simulink model "oving2"  (R2024b)
settings: Solver=ode2  StartTime=0.0  StopTime=100  FixedStep=0.01  RelTol=1e-9  AbsTol=1e-9
values from neighbouring files (symbols this model uses):
  U = 0.5    [oving2_data.m]
  w = 0.3    [oving2_data.m]
  w1 = 0.3    [oving2_data.m]
  w2 = 0.55    [oving2_data.m]
  w3 = 0.8    [oving2_data.m]
undefined symbols (not defined in the file or in its folder): a, b, c, d, f, g, h, i, j, k, l, m, n, o, p
libraries: simulink x17
settings Model: Creator=tormod  LastModifiedBy=john
settings DebuggingCC: UnconnectedInputMsg=warning  UnconnectedOutputMsg=warning  UnconnectedLineMsg=warning
settings ModelReferenceCC: EnableRefExpFcnMdlSchedulingChecks=on
settings RTWCC: GPUComputeCapability=3.5  DLArmComputeVersion=19.05

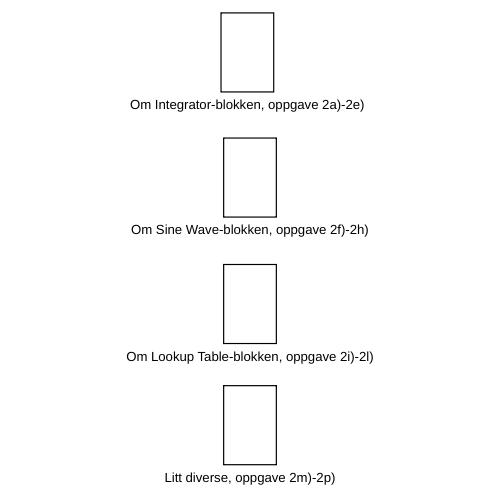
[thumbnail: Simulink's stored preview of the top-level diagram]
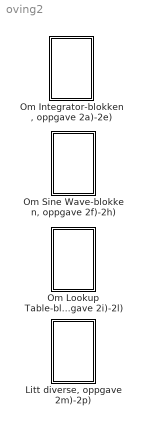
== system oving2 ==
  "Litt diverse, oppgave 2m)-2p)" : Subsystem
  "Om Integrator-blokken, oppgave 2a)-2e)" : Subsystem
  "Om Lookup Table-blokken, oppgave 2i)-2l)" : Subsystem
  "Om Sine Wave-blokken, oppgave 2f)-2h)" : Subsystem

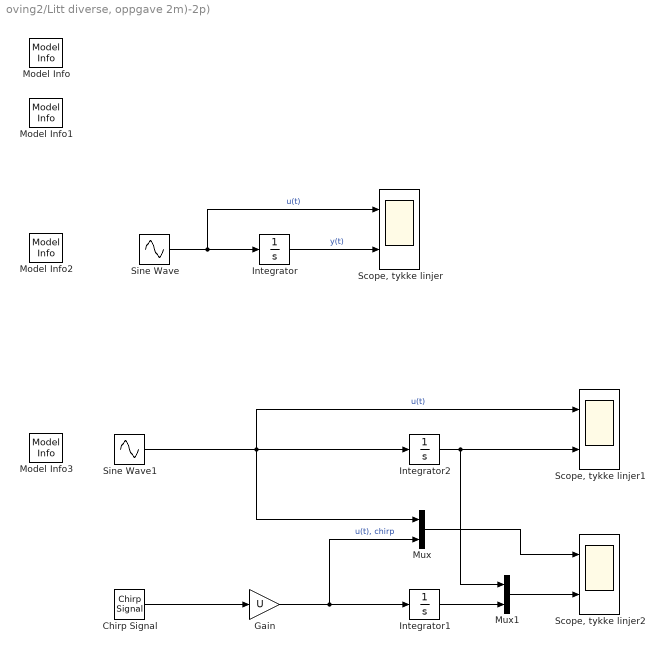
== system oving2/Litt diverse, oppgave 2m)-2p) ==
  Chirp Signal : simulink/Sources/Chirp Signal  f1=f1  T=100  f2=f3
      settings: AttributesFormatString=|
      | u(t) = sin(2 pi f(t) t)
      | f(t) = %<f1> + (%<f2>-%<f1>)/%<T>*t   [Hz]
  Gain : Gain  Gain=U
  Integrator : Integrator  InitialCondition=-5/3
      settings: AttributesFormatString=IC = %<InitialCondition>
  Integrator1 : Integrator  InitialCondition=-U/w1
      settings: AttributesFormatString=IC = %<InitialCondition>
  Integrator2 : Integrator  InitialCondition=[-U/w1, -U/w2, -U/w3]
      settings: AttributesFormatString=IC = %<InitialCondition>
  Model Info : simulink/Model-Wide Utilities/Model Info  Frame=on  DisplayStringWithTags=m)  HorizontalTextAlignment=Center  LeftAlignmentValue=0.5
  Model Info1 : simulink/Model-Wide Utilities/Model Info  Frame=on  DisplayStringWithTags=n)  HorizontalTextAlignment=Center  LeftAlignmentValue=0.5
  Model Info2 : simulink/Model-Wide Utilities/Model Info  Frame=on  DisplayStringWithTags=o)  HorizontalTextAlignment=Center  LeftAlignmentValue=0.5
  Model Info3 : simulink/Model-Wide Utilities/Model Info  Frame=on  DisplayStringWithTags=p)  HorizontalTextAlignment=Center  LeftAlignmentValue=0.5
  Mux : Mux  Inputs=2
  Mux1 : Mux  Inputs=2
  "Scope, tykke linjer" : Scope  NumInputPorts=2
  "Scope, tykke linjer1" : Scope  NumInputPorts=2
  "Scope, tykke linjer2" : Scope  NumInputPorts=2
  Sine Wave : Sin  Amplitude=U  Frequency=w  SampleTime=0
      settings: AttributesFormatString=u(t) = %<Amplitude> sin(%<Frequency>t + %<Phase>) + %<Bias>
  Sine Wave1 : Sin  Amplitude=U  Frequency=[w1, w2, w3]  SampleTime=0
      settings: AttributesFormatString=u(t) = %<Amplitude> sin(%<Frequency>t + %<Phase>) + %<Bias>
  wires:
  Sine Wave/1 -> "Scope, tykke linjer"/1, Integrator/1  "u(t)"
  Integrator/1 -> "Scope, tykke linjer"/2  "y(t)"
  Chirp Signal/1 -> Gain/1
  Gain/1 -> Integrator1/1, Mux/2  "u(t), chirp"
  Sine Wave1/1 -> "Scope, tykke linjer1"/1, Mux/1, Integrator2/1  "u(t)"
  Integrator2/1 -> Mux1/1, "Scope, tykke linjer1"/2
  Mux1/1 -> "Scope, tykke linjer2"/2
  Integrator1/1 -> Mux1/2
  Mux/1 -> "Scope, tykke linjer2"/1

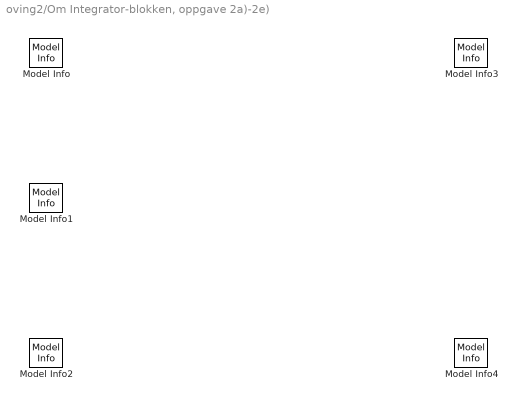
== system oving2/Om Integrator-blokken, oppgave 2a)-2e) ==
  Model Info : simulink/Model-Wide Utilities/Model Info  Frame=on  DisplayStringWithTags=a)  HorizontalTextAlignment=Center  LeftAlignmentValue=0.5
  Model Info1 : simulink/Model-Wide Utilities/Model Info  Frame=on  DisplayStringWithTags=b)  HorizontalTextAlignment=Center  LeftAlignmentValue=0.5
  Model Info2 : simulink/Model-Wide Utilities/Model Info  Frame=on  DisplayStringWithTags=c)  HorizontalTextAlignment=Center  LeftAlignmentValue=0.5
  Model Info3 : simulink/Model-Wide Utilities/Model Info  Frame=on  DisplayStringWithTags=d)  HorizontalTextAlignment=Center  LeftAlignmentValue=0.5
  Model Info4 : simulink/Model-Wide Utilities/Model Info  Frame=on  DisplayStringWithTags=e)  HorizontalTextAlignment=Center  LeftAlignmentValue=0.5

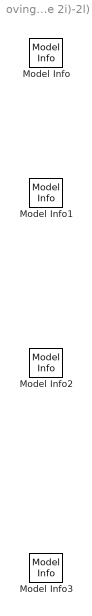
== system oving2/Om Lookup Table-blokken, oppgave 2i)-2l) ==
  Model Info : simulink/Model-Wide Utilities/Model Info  Frame=on  DisplayStringWithTags=i)  HorizontalTextAlignment=Center  LeftAlignmentValue=0.5
  Model Info1 : simulink/Model-Wide Utilities/Model Info  Frame=on  DisplayStringWithTags=j)  HorizontalTextAlignment=Center  LeftAlignmentValue=0.5
  Model Info2 : simulink/Model-Wide Utilities/Model Info  Frame=on  DisplayStringWithTags=k)  HorizontalTextAlignment=Center  LeftAlignmentValue=0.5
  Model Info3 : simulink/Model-Wide Utilities/Model Info  Frame=on  DisplayStringWithTags=l)  HorizontalTextAlignment=Center  LeftAlignmentValue=0.5

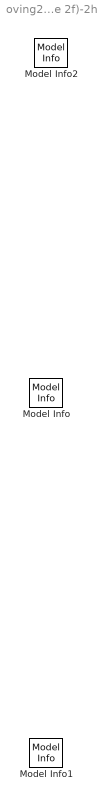
== system oving2/Om Sine Wave-blokken, oppgave 2f)-2h) ==
  Model Info : simulink/Model-Wide Utilities/Model Info  Frame=on  DisplayStringWithTags=g)  HorizontalTextAlignment=Center  LeftAlignmentValue=0.5
  Model Info1 : simulink/Model-Wide Utilities/Model Info  Frame=on  DisplayStringWithTags=h)  HorizontalTextAlignment=Center  LeftAlignmentValue=0.5
  Model Info2 : simulink/Model-Wide Utilities/Model Info  Frame=on  DisplayStringWithTags=f)  HorizontalTextAlignment=Center  LeftAlignmentValue=0.5
